simulink model "case1"  (Simulink 5.0)
settings: Solver=FixedStepDiscrete  StartTime=0.0  StopTime=0.2  FixedStep=Ts  RelTol=1e-4
PreLoadFcn:
  | assignin('base','Ts',[50e-6])
InitFcn:
  | powericon('psbinitsys',bdroot);
undefined symbols (not defined in the file): D1, Delta, Ts
libraries: powerlib2 x69
settings Model: Creator=sybille  LastModifiedBy=pavel  ExtModeTrigMode=oneshot  ExtModeArmWhenConnect=off  LimitDataPoints=off  AlgebraicLoopMsg=none  UnconnectedInputMsg=none  UnconnectedOutputMsg=none  BlockReductionOpt=off  BooleanDataType=off  ProdHWWordLengths=8,32,16,32

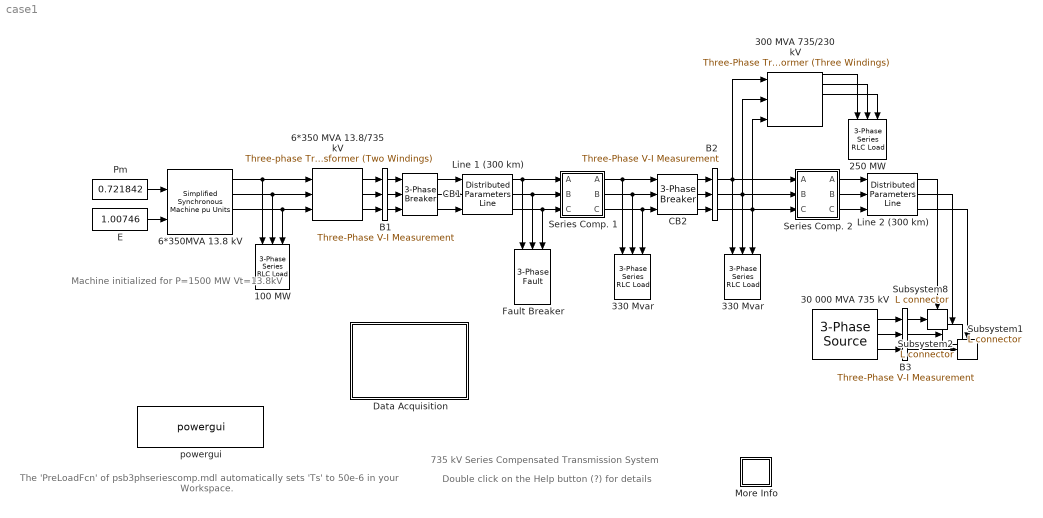
== system case1 ==
  note: Machine initialized for
      |  P=1500 MW Vt=13.8kV
  note: 735 kV Series Compensated Transmission System
  note: Double click on the Help button (?) for details
  note: The 'PreLoadFcn' of psb3phseriescomp.mdl
      | automatically sets 'Ts' to 50e-6 in your Workspace.
  100 MW : powerlib2/Elements/3-Phase Series RLC Load  Orientation=down  Vpp=13.8e3  fn=60  P3=100e6  QL3=0  QC3=0
  250 MW : powerlib2/Elements/3-Phase Series RLC Load  Orientation=down  Vpp=230e3  fn=60  P3=250e6  QL3=0  QC3=0
  30 000 MVA 735 kV : powerlib2/Electrical Sources/3-Phase Source  Tag=PoWeRsYsTeMbLoCk  V=735e3  Phi=0  F=60  InternalConnection=Yg  RLoff=on  R=735^2/30000/10  L=735^2/30000/377  Psc=30000e6  Vbase=735e3  XRratio=10  PSBOutputType=111
  300 MVA 735/230 kV : powerlib2/Elements/Three-Phase Transformer (Three Windings)  Tag=PoWeRsYsTeMbLoCk  confi=ABC as input terminals  nom=[ 300e6 , 60 ]  ydw1=Yg  w1=[ 735e3 , 0.002 , 0.15 ]  ydw2=Yg  w2=[ 230e3 , 0.002 , 0 ]  ydw3=Delta (D1)  w3=[ 25e3 , 0.05 , 0.20 ]  ynsat=on  rmag=500  lm=1000  sat="[  0,0  ;  0.0012,1.2  ;  1.0,1.45 ]"  hyst=off  matfile='hysteresis'  sif=off  ifl=[0.8 -0.8 0.7]  initialslopes=[+1 +1 +1]  mesure=None  PSBOutputType=1111111
  330 Mvar : powerlib2/Elements/3-Phase Series RLC Load  Orientation=down  Vpp=735e3  fn=60  P3=330e6/250  QL3=330e6  QC3=0
  "330 Mvar " : powerlib2/Elements/3-Phase Series RLC Load  Orientation=down  Vpp=735e3  fn=60  P3=330e6/250  QL3=330e6  QC3=0
  6*350 MVA 13.8/735 kV : powerlib2/Elements/Three-phase Transformer (Two Windings)  Tag=PoWeRsYsTeMbLoCk  nominal=[ 6*350e6 , 60 ]  type1=Delta (D1)  params1=[ 13.8e3 , 0.002 , 0.08 ]  type2=Yg  params2=[ 735e3 , 0.002 , 0.08 ]  ynsat=off  rmag=500  lm=500  sat=[ 0,0 ; 0.0024,1.2 ; 1.0,1.52 ]  hyst=off  matfile='hysteresis'  sif=off  phi0=[ 0.8 , -0.8 , 0.7 ]  initialslopes=[+1 +1 +1]  mesure=None  PSBOutputType=111
  6*350MVA 13.8 kV : powerlib2/Machines/Simplified Synchronous  Machine  pu Units  Tag=PoWeRsYsTeMbLoCk  conType=3-wire Y  x1="[ 6*350e6 13.8e3  60 ]"  x2=[ inf,0,2 ]  x3="[ 0.22/15  0.22 ]"  x4=[0 3.29695 0.717757 0.717757 0.717757 -0.0992806 -120.099 119.901]  PSBOutputType=1110  iounits=0  LoadFlowParameters=[1,0,0,0,0]
  B1 : powerlib2/Measurements/Three-Phase V-I Measurement  Tag=PoWeRsYsTeMmEaSuReMeNt  VChoice=phase-to-ground  ualv=on  labelV=Vabc_B1  Vpu=on  Vbase=735e3  IChoice=yes  ualc=on  labelC=Iabc_B1  Ppu=on  Pbase=100e6  OutputType=Complex  PhasorSimulation=off  PSBequivalent=0  PSBOutputType=11100
  B2 : powerlib2/Measurements/Three-Phase V-I Measurement  Tag=PoWeRsYsTeMmEaSuReMeNt  VChoice=phase-to-ground  ualv=on  labelV=Vabc_B2  Vpu=on  Vbase=735e3  IChoice=yes  ualc=on  labelC=Iabc_B2  Ppu=on  Pbase=100e6  OutputType=Complex  PhasorSimulation=off  PSBequivalent=0  PSBOutputType=11100
  B3 : powerlib2/Measurements/Three-Phase V-I Measurement  Tag=PoWeRsYsTeMmEaSuReMeNt  VChoice=no  ualv=off  labelV=Vabc_B3  Vpu=off  Vbase=0  IChoice=no  ualc=off  labelC=Iabc_B3  Ppu=off  Pbase=0  OutputType=Complex  PhasorSimulation=off  PSBequivalent=1  PSBOutputType=11100
  CB1 : powerlib2/Elements/3-Phase Breaker  init_states=closed  sa=on  sb=on  sc=on  sw_times="[5/60  ]"  Ts=Ts  comext=off  Ron=0.001  Rp=1e5  Cp=inf  mesure=None
  CB2 : powerlib2/Elements/3-Phase Breaker  init_states=closed  sa=on  sb=on  sc=on  sw_times="[5/60  ]"  Ts=Ts  comext=off  Ron=0.001  Rp=1e5  Cp=inf  mesure=None
  Data Acquisition : Subsystem
      mask Type: Data Acquisition
      mask Display: disp('Open this block\nto visualize\nrecorded signals')
  E : Constant  Value=1.00746
  Fault Breaker : powerlib2/Elements/3-Phase Fault  Orientation=down  sa=on  sb=on  sc=on  Rdef=0.001  st=on  Rt=1  comext=off  sw_status=[1 0]  sw_times=[ 1/60 6/60]  Ts=Ts  init_statext=[0 0 1]  Rp=inf  Cp=inf  mesure=Fault currents
  Line 1 (300 km) : powerlib2/Elements/Distributed Parameters Line  Tag=PoWeRsYsTeMbLoCk  n=3  f=60  r=[0.01273 0.3864]  l="[0.9337e-3  4.1264e-3]"  c=[12.74e-9 7.751e-9]  lgt=300  x1=[0 -2.475e-008 3.253e+005 -6.709e+005;0.0003733 -2.356e-008 4.162e+005 -6.186e+005;0.0007465 -2.192e-008 4.989e+005 -5.541e+005;0.00112 -1.983e-008 5.716e+005 -4.787e+005;0.001493 -1.736e-008 6.331e+005 -3.938e+005;0.001866 -1.454e-008 6.821e+005 -3.011e+005]  x2=[0 -7.661e-009 1.438e+005 -7.357e+005;0.0003733 -7.194e-009 2.455e+005 -7.083e+005;0.0007465 -6.585e-009 3.424e+005 -6.668e+005;0.00112 -5.846e-009 4.326e+005 -6.122e+005;0.001493 -4.991e-009 5.142e+005 -5.455e+005;0.001866 -4.038e-009 5.856e+005 -4.68e+005]  x3=[0 -1.777e-011 17.22 -960.1;0.0003733 -1.332e-011 151.7 -948.2;0.0007465 -8.607e-012 283.2 -917.5;0.00112 -3.722e-012 409.1 -868.7;0.001493 1.237e-012 526.9 -802.8;0.001866 6.171e-012 634.2 -721]  x4=[0 -2.554e-011 678 -4520;0.0003733 -2.99e-011 1305 -4380;0.0007465 -3.366e-011 1907 -4154;0.00112 -3.676e-011 2470 -3846;0.001493 -3.914e-011 2985 -3461;0.001866 -4.074e-011 3441 -3008]  x5=0.001866  mesure=None  PSBOutputType=111111111111111111111111111111
  Line 2 (300 km) : powerlib2/Elements/Distributed Parameters Line  Tag=PoWeRsYsTeMbLoCk  n=3  f=60  r=[0.01273 0.3864]  l="[0.9337e-3  4.1264e-3]"  c=[12.74e-9 7.751e-9]  lgt=300  x1=[0 -1.083e-008 2.734e+005 -6.876e+005;0.0003733 -1.025e-008 3.672e+005 -6.425e+005;0.0007465 -9.473e-009 4.536e+005 -5.847e+005;0.00112 -8.508e-009 5.311e+005 -5.153e+005;0.001493 -7.375e-009 5.982e+005 -4.357e+005;0.001866 -6.096e-009 6.534e+005 -3.475e+005]  x2=[0 -4.354e-010 1.25e+005 -7.321e+005;0.0003733 -3.901e-010 2.265e+005 -7.074e+005;0.0007465 -3.37e-010 3.235e+005 -6.686e+005;0.00112 -2.773e-010 4.14e+005 -6.166e+005;0.001493 -2.12e-010 4.964e+005 -5.525e+005;0.001866 -1.426e-010 5.69e+005 -4.774e+005]  x3=[0 -4.132e-012 22.32 -1297;0.0003733 -1.462e-012 204 -1281;0.0007465 1.237e-012 381.6 -1240;0.00112 3.912e-012 551.7 -1174;0.001493 6.509e-012 710.8 -1085;0.001866 8.978e-012 855.9 -974.4]  x4=[0 -1.167e-011 405.1 -4181;0.0003733 -1.439e-011 987.4 -4082;0.0007465 -1.682e-011 1550 -3904;0.00112 -1.892e-011 2082 -3648;0.001493 -2.065e-011 2573 -3319;0.001866 -2.197e-011 3013 -2926]  x5=0.001866  mesure=None  PSBOutputType=111111111111111111111111111111
  More Info : Subsystem
      mask Display: disp('?')
  Pm : Constant  Value=0.721842
  Series Comp. 1 : Subsystem
      mask Display: plot(0,0,100,100,[25 45],[50 50], [45 45],[35 65],[55 55],[35 65], [55 75],[50 50])
  Series Comp. 2 : Subsystem
      mask Display: plot(0,0,100,100,[25 45],[50 50], [45 45],[35 65],[55 55],[35 65], [55 75],[50 50])
  Subsystem1 : powerlib2/Connectors/L connector  Tag=PoWeRsYsTeMbLoCk
  Subsystem2 : powerlib2/Connectors/L connector  Tag=PoWeRsYsTeMbLoCk
  Subsystem8 : powerlib2/Connectors/L connector  Tag=PoWeRsYsTeMbLoCk
  powergui : powerlib2/powergui  Frange=0:0.5:500  Ylog=off  Xlog=off  save=on  variable=Zmes  ZoomFFT=on  StartTime=0.0  cycles=1  DisplayStyle=off  fundamental=60  FreqAxis=off  MaxFrequency=1000  frequencyindice=1  frequencyindicesteady=1  RmsSteady=1  display=off  Ts=Ts  methode=off  frequency=60  echomessages=off
  wires:
  B3/1 -> Subsystem8/1
  B3/2 -> Subsystem1/1
  B3/3 -> Subsystem2/1
  6*350 MVA 13.8/735 kV/1 -> B1/1
  6*350 MVA 13.8/735 kV/2 -> B1/2
  6*350 MVA 13.8/735 kV/3 -> B1/3
  6*350MVA 13.8 kV/1 -> 6*350 MVA 13.8/735 kV/1, 100 MW/1
  6*350MVA 13.8 kV/2 -> 6*350 MVA 13.8/735 kV/2, 100 MW/2
  6*350MVA 13.8 kV/3 -> 6*350 MVA 13.8/735 kV/3, 100 MW/3
  Pm/1 -> 6*350MVA 13.8 kV/1
  E/1 -> 6*350MVA 13.8 kV/2
  B1/1 -> CB1/1
  B1/2 -> CB1/2
  B1/3 -> CB1/3
  Line 1 (300 km)/1 -> Series Comp. 1/1(A), Fault Breaker/1
  Line 1 (300 km)/2 -> Series Comp. 1/2(B), Fault Breaker/2
  Line 1 (300 km)/3 -> Series Comp. 1/3(C), Fault Breaker/3
  CB1/1 -> Line 1 (300 km)/1
  CB1/2 -> Line 1 (300 km)/2
  CB1/3 -> Line 1 (300 km)/3
  Series Comp. 1/1("A ") -> CB2/1, 330 Mvar/1
  Series Comp. 1/2("B ") -> CB2/2, 330 Mvar/2
  Series Comp. 1/3("C ") -> CB2/3, 330 Mvar/3
  CB2/1 -> B2/1
  CB2/2 -> B2/2
  CB2/3 -> B2/3
  B2/1 -> Series Comp. 2/1(A), "330 Mvar "/1, 300 MVA 735/230 kV/1
  B2/2 -> Series Comp. 2/2(B), "330 Mvar "/2, 300 MVA 735/230 kV/2
  B2/3 -> "330 Mvar "/3, Series Comp. 2/3(C), 300 MVA 735/230 kV/3
  Series Comp. 2/1("A ") -> Line 2 (300 km)/1
  Series Comp. 2/2("B ") -> Line 2 (300 km)/2
  Series Comp. 2/3("C ") -> Line 2 (300 km)/3
  Line 2 (300 km)/1 -> Subsystem8/Enable
  Line 2 (300 km)/2 -> Subsystem1/Enable
  Line 2 (300 km)/3 -> Subsystem2/Enable
  300 MVA 735/230 kV/1 -> 250 MW/1
  300 MVA 735/230 kV/2 -> 250 MW/2
  300 MVA 735/230 kV/3 -> 250 MW/3
  30 000 MVA 735 kV/1 -> B3/1
  30 000 MVA 735 kV/2 -> B3/2
  30 000 MVA 735 kV/3 -> B3/3

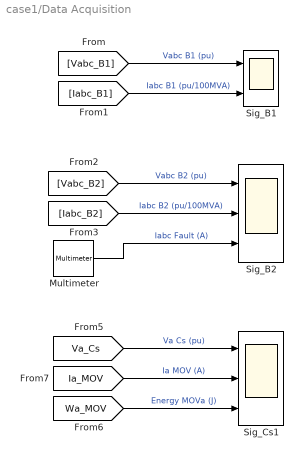
== system case1/Data Acquisition ==
  Multimeter : powerlib2/Measurements/Multimeter  Tag=PoWeRsYsTeMmEaSuReMeNt  PhasorSimulation=off  OutputType=Magnitude  sel=[1 2 3]  L=3  Gain=[1 1 1]  yselected={'Ib: Fault Breaker/Fault A','Ib: Fault Breaker/Fault B','Ib: Fault Breaker/Fault C'};  PSBOutputType=1  PSBequivalent=0  AxesSetting=[0,0.1,-100,100]  Display=0  SavedBlockNames={}
  Sig_B1 : Scope  NumInputPorts=2
      settings: TimeRange=0.2  YMin=-1.5~-20  YMax=1.5~40  SaveName=Sig_B1  SampleInput=on  SampleTime=Ts
  Sig_B2 : Scope  NumInputPorts=3
      settings: TimeRange=0.2  YMin=-2~-100~-10000  YMax=4~100~20000  SaveName=Sig_B2  SampleInput=on  SampleTime=Ts
  Sig_Cs1 : Scope  NumInputPorts=3
      settings: TimeRange=0.2  YMin=-300000~-10000~0  YMax=300000~15000~4e+007  SaveName=Sig_Cs1  SampleInput=on  SampleTime=Ts
  wires:
  [Vabc_B1] -> Sig_B1/1  "Vabc B1 (pu)"
  [Iabc_B1] -> Sig_B1/2  "Iabc B1 (pu/100MVA)"
  [Vabc_B2] -> Sig_B2/1  "Vabc B2 (pu)"
  [Iabc_B2] -> Sig_B2/2  "Iabc B2 (pu/100MVA)"
  Multimeter/1 -> Sig_B2/3  "Iabc Fault (A)"
  [Va_Cs] -> Sig_Cs1/1  "Va Cs (pu)"
  [Ia_MOV] -> Sig_Cs1/2  "Ia MOV (A)"
  [Wa_MOV] -> Sig_Cs1/3  "Energy MOVa (J)"

== system case1/More Info ==
  note: G. Sybille (Hydro-Québec)
  note: Demonstration
  note: This demonstration ilustrates use of  three-phase blocks
      | to study transients on a series-compensated 735-kV transmission system
  note: Circuit Description
  note: Fault and line switching:
  note: A three-phase, 60 Hz, 735 kV power system transmitting power from a power plant consisting of six 350 MVA generators to an equivalent network through a 600 km
      | transmission line. The transmission line is split in two 300 km lines connected between buses B1,B2, and B3. In order to increase the transmission capacity, each line
      | is series compensated by capacitors representing 40% of the line reactance. Both lines are also shunt compensated by a 330 Mvar shunt reactance. The shunt and series
      | compensation equipments are located at the B2 substation  where a 300 MVA 735/230 kV transformer with a 25 kV tertiary winding feeds a 230 kV, 250 MW load.
      | The series compensation subsystems are identical for the two lines. For each line Each phase containsof the series compensation module contains the series capacitor ,
      | a metal oxide varistor (MOV) protecting the capacitor, and a parallel gap protecting the MOV. When the energy dissipated in the MOV exceeds a threshold level of 30 MJ,
      | the gap simulated by a circuit breaker is fired. CB1 and CB2 are the the two line circuit breakers .
      | The generators are simulated with a Simplified Synchronous Machine block. Universal transformer blocks (two-windings and three-windings) are used to model the two
      | transformers.  Saturation is implemented on the transformer connected at bus B2.  Voltages and currents are measured in B1, B2, and B3 blocks.
      | These blocks are 3-phase V-I Measurement blocks where  voltage and current  signals are sent to the Data Acquisition block through Goto blocks.
  note: You will now study the transient performance of this circuit when a line-to-ground and three-phase-to-ground faults are applied on line 1.
      | The fault and the two line circuit breakers CB1 and CB2  are simulated with blocks from the three-phase library.
      | Open the dialog boxes of CB1 and CB2. See how the initial breaker status and switching times are specified.
      | A line-to-ground fault is applied on phase A at t = 1cycle. The two circuit breakers which are initially closed are then open at t = 5 cycles,
      | simulating a fault detection and opening time of 4 cycles. The fault is eliminated at t = 6 cycles, one cycle after line opening.
  note: Notice that this system contains the Discrete System block.  In addition, when you open the system the 'psb3phaseseriescomp' system, the  sampling time Ts = 50e-6 is
      | automatically set in your workspace. The system will therefore be discretized using a 50 microseconds sample time.
  note: Double click on the Data Acquisition block and open the three scopes. Start the simulation.  As the system has already been initialized (1500 MW generation at the 13.8 kV bus)
      | with the Lod Flow utility of the Powergui, the simulation starts in steady state. At t = 1 cycle a line-to-ground fault is applied and the fault current reaches 10 kA .
      | During the fault, the MOV conducts at every half cycle and the energy dissipated in the MOV builds up to 13 MJ.
      | At t = 5 cycles the line protection relays (not simulated) open breakers CB1 and CB2 and the energy stays constant at 13 MJ.  As the maximum energy does not exceed
      | the 30 MJ threshold level,  the gap is not fired. After breaker opening the fault current drops to a small value and the line and series capacitance start to discharge through the
      | fault and the shunt reactance. The fault current extinguishes at the first zero crossing after the opening order given to the fault breaker (t = 6 cycles). Then, the series capacitor
      | stops discharging and its voltage oscillates around 220 kV .
  note: Line-to-Ground Fault
  note: Three-Phase-to-Ground Fault
  note: Change the fault type to a three-phase-to-ground fault by checking Phases A,B and C in in the Fault Breaker block.
      | Restart the simulation. Notice that during the fault the energy dissipated in the MOV builds up faster that in the case of a line-to-ground fault.
      | The energy reaches the 30 MJ threshold level after 3 cycles, one cycle before opening of the line breakers.
      | As a result, the gap is fired and the capacitor voltage  quickly discharges to zero through the damping circuit.
  note: Note : This automatic definition of a variable (Ts) is made possible through the PreLoadFcn. Use "get_param(gcs,'PreLoadFcn')" to see how this variable is defined.
  note: (See case study 'Series Compensated Transmission Network' in the SimPowerSystems User's Guide

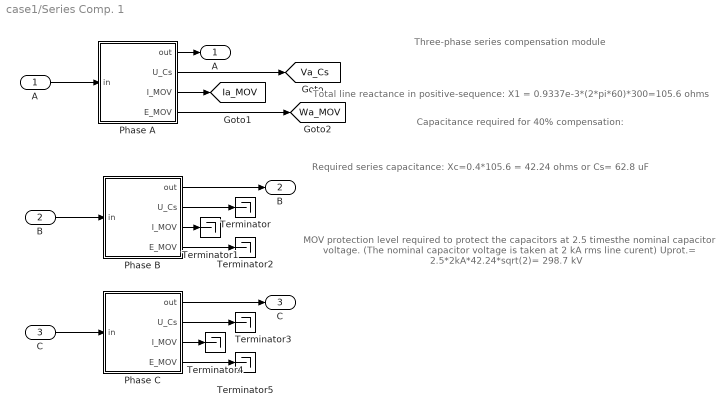
== system case1/Series Comp. 1 ==
  note: Three-phase series compensation module
  note: MOV protection level required to protect the capacitors
      |  at 2.5 timesthe nominal capacitor voltage.
      | (The nominal capacitor voltage is taken at 2 kA  rms line curent)
      |
      | Uprot.= 2.5*2kA*42.24*sqrt(2)= 298.7 kV
  note: Required series capacitance:
      | Xc=0.4*105.6 = 42.24 ohms
      | or Cs= 62.8 uF
  note: Total line reactance in positive-sequence:
      |  X1 = 0.9337e-3*(2*pi*60)*300=105.6 ohms
  note: Capacitance required for 40% compensation:
  A : Inport
  B : Inport  Port=2
  C : Inport  Port=3
  Phase A : Subsystem
  Phase B : Subsystem
  Phase C : Subsystem
  Terminator{,1..5} (6 alike) : Terminator
  "A " : Outport  InitialOutput=0
  "B " : Outport  Port=2  InitialOutput=0
  "C " : Outport  Port=3  InitialOutput=0
  tag scope: Ia_MOV=global, Va_Cs=global, Wa_MOV=global
  wires:
  Phase C/4(E_MOV) -> Terminator5/1
  Phase C/3(I_MOV) -> Terminator4/1
  Phase C/2(U_Cs) -> Terminator3/1
  Phase C/1(out) -> "C "/1
  C/1 -> Phase C/1(in)
  Phase B/4(E_MOV) -> Terminator2/1
  Phase B/3(I_MOV) -> Terminator1/1
  Phase B/2(U_Cs) -> Terminator/1
  Phase B/1(out) -> "B "/1
  B/1 -> Phase B/1(in)
  Phase A/1(out) -> "A "/1
  A/1 -> Phase A/1(in)
  Phase A/2(U_Cs) -> [Va_Cs]
  Phase A/3(I_MOV) -> [Ia_MOV]
  Phase A/4(E_MOV) -> [Wa_MOV]

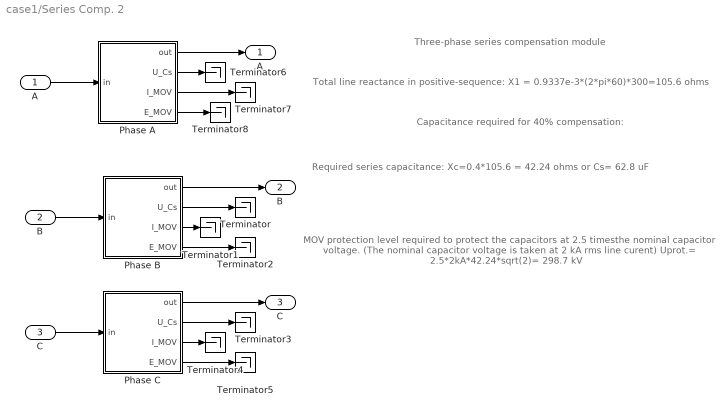
== system case1/Series Comp. 2 ==
  note: Capacitance required for 40% compensation:
  note: Total line reactance in positive-sequence:
      |  X1 = 0.9337e-3*(2*pi*60)*300=105.6 ohms
  note: Required series capacitance:
      | Xc=0.4*105.6 = 42.24 ohms
      | or Cs= 62.8 uF
  note: MOV protection level required to protect the capacitors
      |  at 2.5 timesthe nominal capacitor voltage.
      | (The nominal capacitor voltage is taken at 2 kA  rms line curent)
      |
      | Uprot.= 2.5*2kA*42.24*sqrt(2)= 298.7 kV
  note: Three-phase series compensation module
  A : Inport
  B : Inport  Port=2
  C : Inport  Port=3
  Phase A : Subsystem
  Phase B : Subsystem
  Phase C : Subsystem
  Terminator{,1..8} (9 alike) : Terminator
  "A " : Outport  InitialOutput=0
  "B " : Outport  Port=2  InitialOutput=0
  "C " : Outport  Port=3  InitialOutput=0
  wires:
  A/1 -> Phase A/1(in)
  Phase A/1(out) -> "A "/1
  B/1 -> Phase B/1(in)
  Phase B/1(out) -> "B "/1
  Phase B/2(U_Cs) -> Terminator/1
  Phase B/3(I_MOV) -> Terminator1/1
  Phase B/4(E_MOV) -> Terminator2/1
  C/1 -> Phase C/1(in)
  Phase C/1(out) -> "C "/1
  Phase C/2(U_Cs) -> Terminator3/1
  Phase C/3(I_MOV) -> Terminator4/1
  Phase C/4(E_MOV) -> Terminator5/1
  Phase A/2(U_Cs) -> Terminator6/1
  Phase A/3(I_MOV) -> Terminator7/1
  Phase A/4(E_MOV) -> Terminator8/1

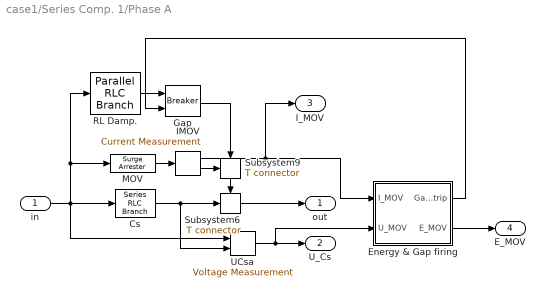
== system case1/Series Comp. 1/Phase A ==
  in : Inport
  Cs : powerlib2/Elements/Series RLC Branch  Tag=PoWeRsYsTeMbLoCk  a=0  b=0  c=62.8e-6  mesure=None  PSBOutputType=1
  Energy & Gap firing : Subsystem
  Gap : powerlib2/Elements/Breaker  Tag=PoWeRsYsTeMbLoCk  a=0.001  c=0  rs=inf  cs=0  times="[ 4/60  5/60 ]"  Ts=0  comext=on  mesure=None  PSBOutputType=1
  IMOV : powerlib2/Measurements/Current Measurement  Tag=PoWeRsYsTeMmEaSuReMeNt  PhasorSimulation=off  OutputType=Magnitude  PSBOutputType=01  PSBequivalent=0
  MOV : powerlib2/Elements/Surge Arrester  Tag=PoWeRsYsTeMbLoCk  x1=298.7e+03  x2=60  x3=500  x4=[.955 50]  x5=[1.0 25]  x6=[.9915 16.5]  mesure=None  PSBOutputType=1
  RL Damp. : powerlib2/Elements/Parallel RLC Branch  Tag=PoWeRsYsTeMbLoCk  a=7.5  b=1.7e-3  c=0  mesure=None  PSBOutputType=1
  Subsystem6 : powerlib2/Connectors/T connector  Tag=PoWeRsYsTeMbLoCk  PSBOutputType=1
  Subsystem9 : powerlib2/Connectors/T connector  Tag=PoWeRsYsTeMbLoCk  Orientation=down  PSBOutputType=1
  UCsa : powerlib2/Measurements/Voltage Measurement  Tag=PoWeRsYsTeMmEaSuReMeNt  PhasorSimulation=off  OutputType=Magnitude  PSBOutputType=0  PSBequivalent=0
  out : Outport
  U_Cs : Outport  Port=2
  I_MOV : Outport  Port=3
  E_MOV : Outport  Port=4
  wires:
  MOV/1 -> IMOV/1
  IMOV/1 -> I_MOV/1, Energy & Gap firing/1(I_MOV)
  Subsystem6/1 -> out/1
  Energy & Gap firing/2(E_MOV) -> E_MOV/1
  UCsa/1 -> U_Cs/1, Energy & Gap firing/2(U_MOV)
  in/1 -> RL Damp./1, MOV/1, Cs/1, UCsa/1
  Cs/1 -> Subsystem6/1, UCsa/2
  Energy & Gap firing/1(Gap_trip) -> Gap/2
  Gap/1 -> Subsystem9/1
  RL Damp./1 -> Gap/1
  Subsystem9/1 -> Subsystem6/Enable
  IMOV/2 -> Subsystem9/Enable

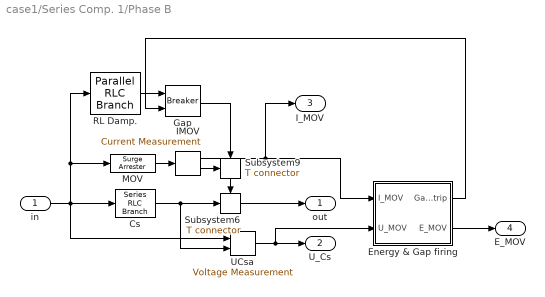
== system case1/Series Comp. 1/Phase B ==
  in : Inport
  Cs : powerlib2/Elements/Series RLC Branch  Tag=PoWeRsYsTeMbLoCk  a=0  b=0  c=62.8e-6  mesure=None  PSBOutputType=1
  Energy & Gap firing : Subsystem
  Gap : powerlib2/Elements/Breaker  Tag=PoWeRsYsTeMbLoCk  a=0.001  c=0  rs=inf  cs=0  times="[ 4/60  5/60 ]"  Ts=0  comext=on  mesure=None  PSBOutputType=1
  IMOV : powerlib2/Measurements/Current Measurement  Tag=PoWeRsYsTeMmEaSuReMeNt  PhasorSimulation=off  OutputType=Magnitude  PSBOutputType=01  PSBequivalent=0
  MOV : powerlib2/Elements/Surge Arrester  Tag=PoWeRsYsTeMbLoCk  x1=298.7e+03  x2=60  x3=500  x4=[.955 50]  x5=[1.0 25]  x6=[.9915 16.5]  mesure=None  PSBOutputType=1
  RL Damp. : powerlib2/Elements/Parallel RLC Branch  Tag=PoWeRsYsTeMbLoCk  a=7.5  b=1.7e-3  c=0  mesure=None  PSBOutputType=1
  Subsystem6 : powerlib2/Connectors/T connector  Tag=PoWeRsYsTeMbLoCk  PSBOutputType=1
  Subsystem9 : powerlib2/Connectors/T connector  Tag=PoWeRsYsTeMbLoCk  Orientation=down  PSBOutputType=1
  UCsa : powerlib2/Measurements/Voltage Measurement  Tag=PoWeRsYsTeMmEaSuReMeNt  PhasorSimulation=off  OutputType=Magnitude  PSBOutputType=0  PSBequivalent=0
  out : Outport
  U_Cs : Outport  Port=2
  I_MOV : Outport  Port=3
  E_MOV : Outport  Port=4
  wires:
  IMOV/2 -> Subsystem9/Enable
  Subsystem9/1 -> Subsystem6/Enable
  RL Damp./1 -> Gap/1
  Gap/1 -> Subsystem9/1
  Energy & Gap firing/1(Gap_trip) -> Gap/2
  Cs/1 -> UCsa/2, Subsystem6/1
  in/1 -> UCsa/1, Cs/1, MOV/1, RL Damp./1
  UCsa/1 -> Energy & Gap firing/2(U_MOV), U_Cs/1
  Energy & Gap firing/2(E_MOV) -> E_MOV/1
  Subsystem6/1 -> out/1
  IMOV/1 -> Energy & Gap firing/1(I_MOV), I_MOV/1
  MOV/1 -> IMOV/1

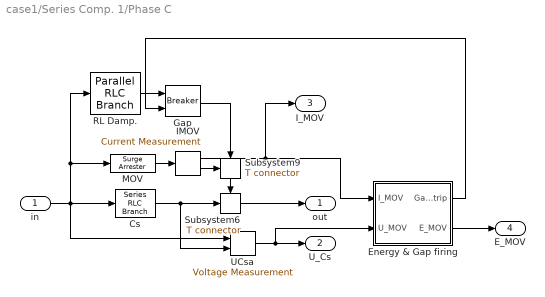
== system case1/Series Comp. 1/Phase C ==
  in : Inport
  Cs : powerlib2/Elements/Series RLC Branch  Tag=PoWeRsYsTeMbLoCk  a=0  b=0  c=62.8e-6  mesure=None  PSBOutputType=1
  Energy & Gap firing : Subsystem
  Gap : powerlib2/Elements/Breaker  Tag=PoWeRsYsTeMbLoCk  a=0.001  c=0  rs=inf  cs=0  times="[ 4/60  5/60 ]"  Ts=0  comext=on  mesure=None  PSBOutputType=1
  IMOV : powerlib2/Measurements/Current Measurement  Tag=PoWeRsYsTeMmEaSuReMeNt  PhasorSimulation=off  OutputType=Magnitude  PSBOutputType=01  PSBequivalent=0
  MOV : powerlib2/Elements/Surge Arrester  Tag=PoWeRsYsTeMbLoCk  x1=298.7e+03  x2=60  x3=500  x4=[.955 50]  x5=[1.0 25]  x6=[.9915 16.5]  mesure=None  PSBOutputType=1
  RL Damp. : powerlib2/Elements/Parallel RLC Branch  Tag=PoWeRsYsTeMbLoCk  a=7.5  b=1.7e-3  c=0  mesure=None  PSBOutputType=1
  Subsystem6 : powerlib2/Connectors/T connector  Tag=PoWeRsYsTeMbLoCk  PSBOutputType=1
  Subsystem9 : powerlib2/Connectors/T connector  Tag=PoWeRsYsTeMbLoCk  Orientation=down  PSBOutputType=1
  UCsa : powerlib2/Measurements/Voltage Measurement  Tag=PoWeRsYsTeMmEaSuReMeNt  PhasorSimulation=off  OutputType=Magnitude  PSBOutputType=0  PSBequivalent=0
  out : Outport
  U_Cs : Outport  Port=2
  I_MOV : Outport  Port=3
  E_MOV : Outport  Port=4
  wires:
  MOV/1 -> IMOV/1
  IMOV/1 -> I_MOV/1, Energy & Gap firing/1(I_MOV)
  Subsystem6/1 -> out/1
  Energy & Gap firing/2(E_MOV) -> E_MOV/1
  UCsa/1 -> U_Cs/1, Energy & Gap firing/2(U_MOV)
  in/1 -> RL Damp./1, MOV/1, Cs/1, UCsa/1
  Cs/1 -> Subsystem6/1, UCsa/2
  Energy & Gap firing/1(Gap_trip) -> Gap/2
  Gap/1 -> Subsystem9/1
  RL Damp./1 -> Gap/1
  Subsystem9/1 -> Subsystem6/Enable
  IMOV/2 -> Subsystem9/Enable

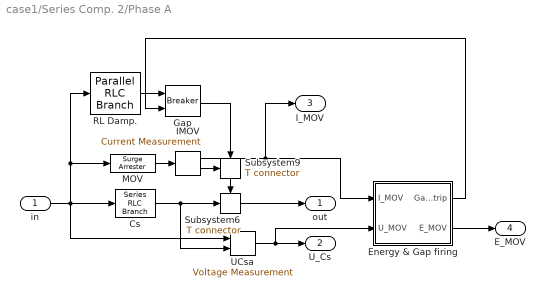
== system case1/Series Comp. 2/Phase A ==
  in : Inport
  Cs : powerlib2/Elements/Series RLC Branch  Tag=PoWeRsYsTeMbLoCk  a=0  b=0  c=62.8e-6  mesure=None  PSBOutputType=1
  Energy & Gap firing : Subsystem
  Gap : powerlib2/Elements/Breaker  Tag=PoWeRsYsTeMbLoCk  a=0.001  c=0  rs=inf  cs=0  times="[ 4/60  5/60 ]"  Ts=0  comext=on  mesure=None  PSBOutputType=1
  IMOV : powerlib2/Measurements/Current Measurement  Tag=PoWeRsYsTeMmEaSuReMeNt  PhasorSimulation=off  OutputType=Magnitude  PSBOutputType=01  PSBequivalent=0
  MOV : powerlib2/Elements/Surge Arrester  Tag=PoWeRsYsTeMbLoCk  x1=298.7e+03  x2=60  x3=500  x4=[.955 50]  x5=[1.0 25]  x6=[.9915 16.5]  mesure=None  PSBOutputType=1
  RL Damp. : powerlib2/Elements/Parallel RLC Branch  Tag=PoWeRsYsTeMbLoCk  a=7.5  b=1.7e-3  c=0  mesure=None  PSBOutputType=1
  Subsystem6 : powerlib2/Connectors/T connector  Tag=PoWeRsYsTeMbLoCk  PSBOutputType=1
  Subsystem9 : powerlib2/Connectors/T connector  Tag=PoWeRsYsTeMbLoCk  Orientation=down  PSBOutputType=1
  UCsa : powerlib2/Measurements/Voltage Measurement  Tag=PoWeRsYsTeMmEaSuReMeNt  PhasorSimulation=off  OutputType=Magnitude  PSBOutputType=0  PSBequivalent=0
  out : Outport
  U_Cs : Outport  Port=2
  I_MOV : Outport  Port=3
  E_MOV : Outport  Port=4
  wires:
  IMOV/2 -> Subsystem9/Enable
  Subsystem9/1 -> Subsystem6/Enable
  RL Damp./1 -> Gap/1
  Gap/1 -> Subsystem9/1
  Energy & Gap firing/1(Gap_trip) -> Gap/2
  Cs/1 -> UCsa/2, Subsystem6/1
  in/1 -> UCsa/1, Cs/1, MOV/1, RL Damp./1
  UCsa/1 -> Energy & Gap firing/2(U_MOV), U_Cs/1
  Energy & Gap firing/2(E_MOV) -> E_MOV/1
  Subsystem6/1 -> out/1
  IMOV/1 -> Energy & Gap firing/1(I_MOV), I_MOV/1
  MOV/1 -> IMOV/1

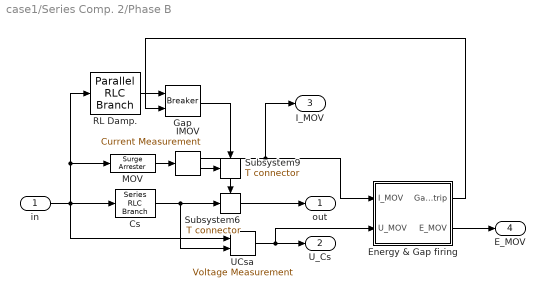
== system case1/Series Comp. 2/Phase B ==
  in : Inport
  Cs : powerlib2/Elements/Series RLC Branch  Tag=PoWeRsYsTeMbLoCk  a=0  b=0  c=62.8e-6  mesure=None  PSBOutputType=1
  Energy & Gap firing : Subsystem
  Gap : powerlib2/Elements/Breaker  Tag=PoWeRsYsTeMbLoCk  a=0.001  c=0  rs=inf  cs=0  times="[ 4/60  5/60 ]"  Ts=0  comext=on  mesure=None  PSBOutputType=1
  IMOV : powerlib2/Measurements/Current Measurement  Tag=PoWeRsYsTeMmEaSuReMeNt  PhasorSimulation=off  OutputType=Magnitude  PSBOutputType=01  PSBequivalent=0
  MOV : powerlib2/Elements/Surge Arrester  Tag=PoWeRsYsTeMbLoCk  x1=298.7e+03  x2=60  x3=500  x4=[.955 50]  x5=[1.0 25]  x6=[.9915 16.5]  mesure=None  PSBOutputType=1
  RL Damp. : powerlib2/Elements/Parallel RLC Branch  Tag=PoWeRsYsTeMbLoCk  a=7.5  b=1.7e-3  c=0  mesure=None  PSBOutputType=1
  Subsystem6 : powerlib2/Connectors/T connector  Tag=PoWeRsYsTeMbLoCk  PSBOutputType=1
  Subsystem9 : powerlib2/Connectors/T connector  Tag=PoWeRsYsTeMbLoCk  Orientation=down  PSBOutputType=1
  UCsa : powerlib2/Measurements/Voltage Measurement  Tag=PoWeRsYsTeMmEaSuReMeNt  PhasorSimulation=off  OutputType=Magnitude  PSBOutputType=0  PSBequivalent=0
  out : Outport
  U_Cs : Outport  Port=2
  I_MOV : Outport  Port=3
  E_MOV : Outport  Port=4
  wires:
  MOV/1 -> IMOV/1
  IMOV/1 -> I_MOV/1, Energy & Gap firing/1(I_MOV)
  Subsystem6/1 -> out/1
  Energy & Gap firing/2(E_MOV) -> E_MOV/1
  UCsa/1 -> U_Cs/1, Energy & Gap firing/2(U_MOV)
  in/1 -> RL Damp./1, MOV/1, Cs/1, UCsa/1
  Cs/1 -> Subsystem6/1, UCsa/2
  Energy & Gap firing/1(Gap_trip) -> Gap/2
  Gap/1 -> Subsystem9/1
  RL Damp./1 -> Gap/1
  Subsystem9/1 -> Subsystem6/Enable
  IMOV/2 -> Subsystem9/Enable

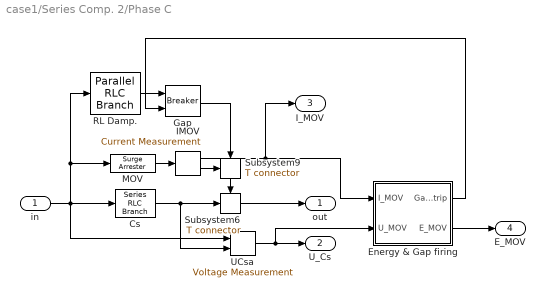
== system case1/Series Comp. 2/Phase C ==
  in : Inport
  Cs : powerlib2/Elements/Series RLC Branch  Tag=PoWeRsYsTeMbLoCk  a=0  b=0  c=62.8e-6  mesure=None  PSBOutputType=1
  Energy & Gap firing : Subsystem
  Gap : powerlib2/Elements/Breaker  Tag=PoWeRsYsTeMbLoCk  a=0.001  c=0  rs=inf  cs=0  times="[ 4/60  5/60 ]"  Ts=0  comext=on  mesure=None  PSBOutputType=1
  IMOV : powerlib2/Measurements/Current Measurement  Tag=PoWeRsYsTeMmEaSuReMeNt  PhasorSimulation=off  OutputType=Magnitude  PSBOutputType=01  PSBequivalent=0
  MOV : powerlib2/Elements/Surge Arrester  Tag=PoWeRsYsTeMbLoCk  x1=298.7e+03  x2=60  x3=500  x4=[.955 50]  x5=[1.0 25]  x6=[.9915 16.5]  mesure=None  PSBOutputType=1
  RL Damp. : powerlib2/Elements/Parallel RLC Branch  Tag=PoWeRsYsTeMbLoCk  a=7.5  b=1.7e-3  c=0  mesure=None  PSBOutputType=1
  Subsystem6 : powerlib2/Connectors/T connector  Tag=PoWeRsYsTeMbLoCk  PSBOutputType=1
  Subsystem9 : powerlib2/Connectors/T connector  Tag=PoWeRsYsTeMbLoCk  Orientation=down  PSBOutputType=1
  UCsa : powerlib2/Measurements/Voltage Measurement  Tag=PoWeRsYsTeMmEaSuReMeNt  PhasorSimulation=off  OutputType=Magnitude  PSBOutputType=0  PSBequivalent=0
  out : Outport
  U_Cs : Outport  Port=2
  I_MOV : Outport  Port=3
  E_MOV : Outport  Port=4
  wires:
  IMOV/2 -> Subsystem9/Enable
  Subsystem9/1 -> Subsystem6/Enable
  RL Damp./1 -> Gap/1
  Gap/1 -> Subsystem9/1
  Energy & Gap firing/1(Gap_trip) -> Gap/2
  Cs/1 -> UCsa/2, Subsystem6/1
  in/1 -> UCsa/1, Cs/1, MOV/1, RL Damp./1
  UCsa/1 -> Energy & Gap firing/2(U_MOV), U_Cs/1
  Energy & Gap firing/2(E_MOV) -> E_MOV/1
  Subsystem6/1 -> out/1
  IMOV/1 -> Energy & Gap firing/1(I_MOV), I_MOV/1
  MOV/1 -> IMOV/1

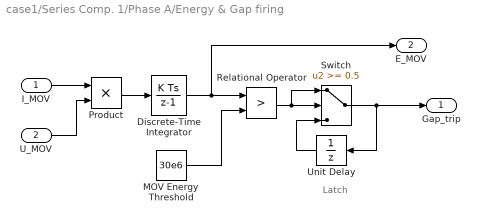
== system case1/Series Comp. 1/Phase A/Energy & Gap firing ==
  note: Latch
  I_MOV : Inport
  U_MOV : Inport  Port=2
  Discrete-Time Integrator : DiscreteIntegrator  SampleTime=Ts
  MOV Energy Threshold : Constant  Value=30e6
  Product : Product  SaturateOnIntegerOverflow=on  InputSameDT=on
  Relational Operator : RelationalOperator  Operator=>  ZeroCross=off  InputSameDT=on
  Switch : Switch  Threshold=0.5  ZeroCross=off  InputSameDT=on
  Unit Delay : UnitDelay  Orientation=left  SampleTime=Ts
  Gap_trip : Outport
  E_MOV : Outport  Port=2  InitialOutput=0
  wires:
  Switch/1 -> Unit Delay/1, Gap_trip/1
  U_MOV/1 -> Product/2
  MOV Energy Threshold/1 -> Relational Operator/2
  Product/1 -> Discrete-Time Integrator/1
  I_MOV/1 -> Product/1
  Discrete-Time Integrator/1 -> E_MOV/1, Relational Operator/1
  Relational Operator/1 -> Switch/1, Switch/2
  Unit Delay/1 -> Switch/3

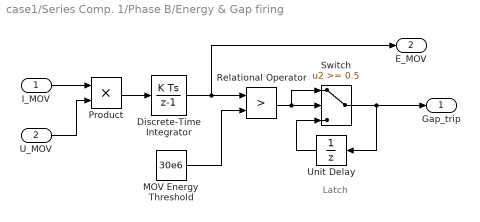
== system case1/Series Comp. 1/Phase B/Energy & Gap firing ==
  note: Latch
  I_MOV : Inport
  U_MOV : Inport  Port=2
  Discrete-Time Integrator : DiscreteIntegrator  SampleTime=Ts
  MOV Energy Threshold : Constant  Value=30e6
  Product : Product  SaturateOnIntegerOverflow=on  InputSameDT=on
  Relational Operator : RelationalOperator  Operator=>  ZeroCross=off  InputSameDT=on
  Switch : Switch  Threshold=0.5  ZeroCross=off  InputSameDT=on
  Unit Delay : UnitDelay  Orientation=left  SampleTime=Ts
  Gap_trip : Outport
  E_MOV : Outport  Port=2  InitialOutput=0
  wires:
  Unit Delay/1 -> Switch/3
  Relational Operator/1 -> Switch/2, Switch/1
  Discrete-Time Integrator/1 -> Relational Operator/1, E_MOV/1
  I_MOV/1 -> Product/1
  Product/1 -> Discrete-Time Integrator/1
  MOV Energy Threshold/1 -> Relational Operator/2
  U_MOV/1 -> Product/2
  Switch/1 -> Gap_trip/1, Unit Delay/1

== system case1/Series Comp. 1/Phase C/Energy & Gap firing ==
  note: Latch
  I_MOV : Inport
  U_MOV : Inport  Port=2
  Discrete-Time Integrator : DiscreteIntegrator  SampleTime=Ts
  MOV Energy Threshold : Constant  Value=30e6
  Product : Product  SaturateOnIntegerOverflow=on  InputSameDT=on
  Relational Operator : RelationalOperator  Operator=>  ZeroCross=off  InputSameDT=on
  Switch : Switch  Threshold=0.5  ZeroCross=off  InputSameDT=on
  Unit Delay : UnitDelay  Orientation=left  SampleTime=Ts
  Gap_trip : Outport
  E_MOV : Outport  Port=2  InitialOutput=0
  wires:
  Switch/1 -> Unit Delay/1, Gap_trip/1
  U_MOV/1 -> Product/2
  MOV Energy Threshold/1 -> Relational Operator/2
  Product/1 -> Discrete-Time Integrator/1
  I_MOV/1 -> Product/1
  Discrete-Time Integrator/1 -> E_MOV/1, Relational Operator/1
  Relational Operator/1 -> Switch/1, Switch/2
  Unit Delay/1 -> Switch/3

== system case1/Series Comp. 2/Phase A/Energy & Gap firing ==
  note: Latch
  I_MOV : Inport
  U_MOV : Inport  Port=2
  Discrete-Time Integrator : DiscreteIntegrator  SampleTime=Ts
  MOV Energy Threshold : Constant  Value=30e6
  Product : Product  SaturateOnIntegerOverflow=on  InputSameDT=on
  Relational Operator : RelationalOperator  Operator=>  ZeroCross=off  InputSameDT=on
  Switch : Switch  Threshold=0.5  ZeroCross=off  InputSameDT=on
  Unit Delay : UnitDelay  Orientation=left  SampleTime=Ts
  Gap_trip : Outport
  E_MOV : Outport  Port=2  InitialOutput=0
  wires:
  Unit Delay/1 -> Switch/3
  Relational Operator/1 -> Switch/2, Switch/1
  Discrete-Time Integrator/1 -> Relational Operator/1, E_MOV/1
  I_MOV/1 -> Product/1
  Product/1 -> Discrete-Time Integrator/1
  MOV Energy Threshold/1 -> Relational Operator/2
  U_MOV/1 -> Product/2
  Switch/1 -> Gap_trip/1, Unit Delay/1

== system case1/Series Comp. 2/Phase B/Energy & Gap firing ==
  note: Latch
  I_MOV : Inport
  U_MOV : Inport  Port=2
  Discrete-Time Integrator : DiscreteIntegrator  SampleTime=Ts
  MOV Energy Threshold : Constant  Value=30e6
  Product : Product  SaturateOnIntegerOverflow=on  InputSameDT=on
  Relational Operator : RelationalOperator  Operator=>  ZeroCross=off  InputSameDT=on
  Switch : Switch  Threshold=0.5  ZeroCross=off  InputSameDT=on
  Unit Delay : UnitDelay  Orientation=left  SampleTime=Ts
  Gap_trip : Outport
  E_MOV : Outport  Port=2  InitialOutput=0
  wires:
  Switch/1 -> Unit Delay/1, Gap_trip/1
  U_MOV/1 -> Product/2
  MOV Energy Threshold/1 -> Relational Operator/2
  Product/1 -> Discrete-Time Integrator/1
  I_MOV/1 -> Product/1
  Discrete-Time Integrator/1 -> E_MOV/1, Relational Operator/1
  Relational Operator/1 -> Switch/1, Switch/2
  Unit Delay/1 -> Switch/3

== system case1/Series Comp. 2/Phase C/Energy & Gap firing ==
  note: Latch
  I_MOV : Inport
  U_MOV : Inport  Port=2
  Discrete-Time Integrator : DiscreteIntegrator  SampleTime=Ts
  MOV Energy Threshold : Constant  Value=30e6
  Product : Product  SaturateOnIntegerOverflow=on  InputSameDT=on
  Relational Operator : RelationalOperator  Operator=>  ZeroCross=off  InputSameDT=on
  Switch : Switch  Threshold=0.5  ZeroCross=off  InputSameDT=on
  Unit Delay : UnitDelay  Orientation=left  SampleTime=Ts
  Gap_trip : Outport
  E_MOV : Outport  Port=2  InitialOutput=0
  wires:
  Unit Delay/1 -> Switch/3
  Relational Operator/1 -> Switch/2, Switch/1
  Discrete-Time Integrator/1 -> Relational Operator/1, E_MOV/1
  I_MOV/1 -> Product/1
  Product/1 -> Discrete-Time Integrator/1
  MOV Energy Threshold/1 -> Relational Operator/2
  U_MOV/1 -> Product/2
  Switch/1 -> Gap_trip/1, Unit Delay/1
